simulink model "MassSpringDamperSystemSim"  (R2022b)
settings: Solver=VariableStepAuto  StartTime=0.0  StopTime=5  MaxStep=.0001  RelTol=1e-3
values from neighbouring files (symbols this model uses):
  b = 10    [MassSpringDamperSystemInit.m]
  k = 400    [MassSpringDamperSystemInit.m]
  m = massValues(i)    [MassSpringDamperSystemInit.m]
  x0 = 1    [MassSpringDamperSystemInit.m]
settings Model: Creator=MOHAMED  LastModifiedBy=MOHAMED

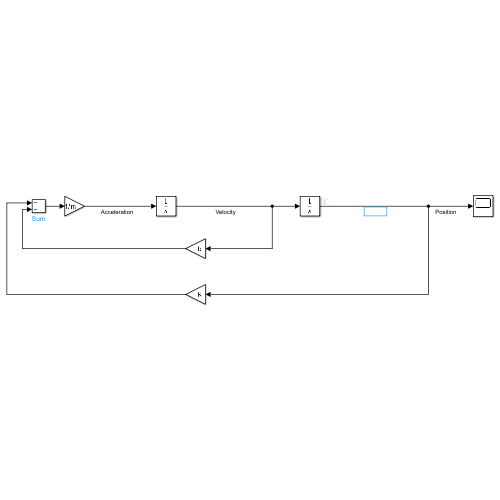
[thumbnail: Simulink's stored preview of the top-level diagram]
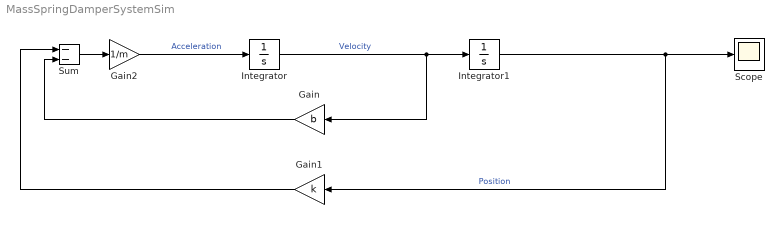
== system MassSpringDamperSystemSim ==
  Gain : Gain  Gain=b
  Gain1 : Gain  Gain=k
  Gain2 : Gain  Gain=1/m
  Integrator : Integrator
  Integrator1 : Integrator  InitialCondition=x0
  Scope : Scope
  Sum : Sum  Inputs=--
  wires:
  Sum/1 -> Gain2/1
  Integrator/1 -> Gain/1, Integrator1/1  "Velocity"
  Integrator1/1 -> Scope/1, Gain1/1  "Position"
  Gain/1 -> Sum/2
  Gain1/1 -> Sum/1
  Gain2/1 -> Integrator/1  "Acceleration"
